simulink model "DOO"  (R2020a)
settings: Solver=FixedStepAuto  StartTime=0.0  StopTime=10.0  FixedStep=1e-3  RelTol=1e-3  EnableMultiTasking=on
settings Model: ExtModeTrigDuration=5  Creator=theodor  LastModifiedBy=theodor
settings OptimizationCC: EnhancedBackFolding=on  PassReuseOutputArgsAs=Individual arguments  ZeroExternalMemoryAtStartup=off  ZeroInternalMemoryAtStartup=off  MaxStackSize=64  OptimizeBlockOrder=speed  DifferentSizesBufferReuse=on  OptimizationCustomize=off  EfficientTunableParamExpr=on
settings DebuggingCC: ParameterTunabilityLossMsg=error
settings HardwareCC: ProdBitPerPointer=32  ProdBitPerSizeT=32  ProdBitPerPtrDiffT=32  ProdLargestAtomicInteger=Long  ProdLargestAtomicFloat=Double  ProdWordSize=32  ProdHWDeviceType=ARM Compatible->ARM Cortex
settings SFSimCC: MATLABDynamicMemAlloc=off
settings RTWCC: SystemTargetFile=ert.tlc  HardwareBoard=NXP FRDM-K64F  TemplateMakefile=ert_default_tmf  Toolchain=GNU Tools for ARM Embedded Processors
settings CodeAppCC: ForceParamTrailComments=on  IgnoreCustomStorageClasses=off  OperatorAnnotations=on  SimulinkDataObjDesc=on  SFDataObjDesc=on  InsertBlockDesc=on

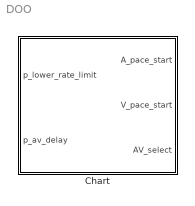
== system DOO ==
  Chart : Stateflow chart  TreatAsAtomicUnit=on

== stateflow chart DOO/Chart ==
  state PACE_VENT
    entry:
    V_pace_start = 1;
    on after(1, msec):
    V_pace_start = 0;
    AV_select = 0;
  state PACE_ATR
    entry:
    A_pace_start = 1;
    on after(1, msec):
    A_pace_start = 0;
    AV_select = 1;
  (default) -> PACE_VENT
  PACE_VENT -> PACE_ATR : after(p_lower_rate_limit - p_av_delay, msec)
  PACE_ATR -> PACE_VENT : after(p_av_delay, msec)
  data: p_lower_rate_limit input; p_av_delay input; A_pace_start output; V_pace_start output; AV_select output
